simulink model "hybrid_controller_old3"  (R2024b)
settings: Solver=VariableStepAuto  StartTime=0.0  StopTime=20  RelTol=1e-3
undefined symbols (not defined in the file or in its folder): extractTop2x2, non_linear_m, non_linear_vcfg, wall_surface
libraries: roblocks x10

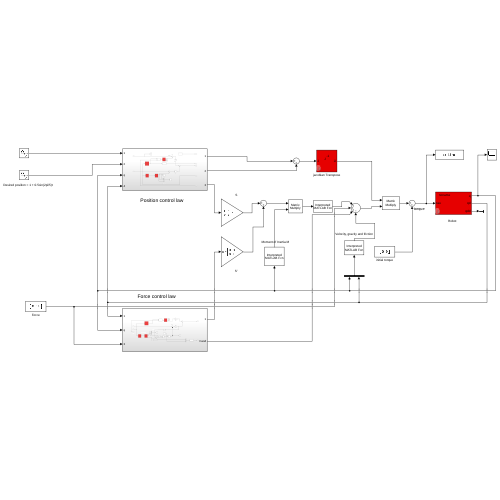
[thumbnail: Simulink's stored preview of the top-level diagram]
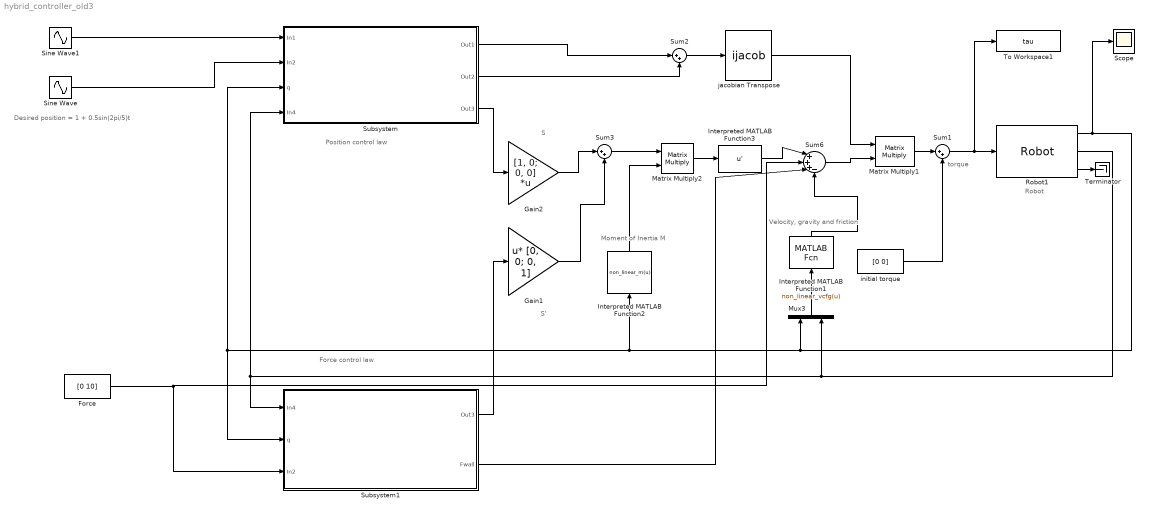
== system hybrid_controller_old3 ==
  note: Robot
  note: S
  note: Desired position = 1 + 0.5sin(2pi/5)t
  note: Position control law
  note: Moment of Inertia M
  note: Velocity, gravity and friction
  note: torque
  note: S'
  note: Force control law
  Force : Constant  Value=[0 10]
  Gain1 : Gain  Gain=[0, 0; 0, 1]  Multiplication=Matrix(u*K)
  Gain2 : Gain  Gain=[1, 0; 0, 0]  Multiplication=Matrix(K*u)
  Interpreted MATLAB Function1 : MATLABFcn  MATLABFcn=non_linear_vcfg(u)  OutputDimensions=[2 1]  Output1D=off
  Interpreted MATLAB Function2 : MATLABFcn  MATLABFcn=non_linear_m(u)  OutputDimensions=[2 2]  Output1D=off
  Interpreted MATLAB Function3 : MATLABFcn  MATLABFcn=u'  OutputDimensions=[2 1]  Output1D=off
  Matrix Multiply1 : Product  Multiplication=Matrix(*)
  Matrix Multiply2 : Product  Multiplication=Matrix(*)
  Mux3 : Mux  Inputs=2
  Robot1 : roblocks/Robot  robot=robot  q0=[0 0 0 0 0 0]
      link override Integrator: InitialCondition=[1 1]
      link override Integrator1: InitialCondition=[1 1]
  Scope : Scope
  Sine Wave : Sin  Amplitude=0.5  Bias=2.2  Frequency=1.256  SampleTime=0
  Sine Wave1 : Sin  Amplitude=0.28  Frequency=1.256  SampleTime=0
  Subsystem : Subsystem
  Subsystem1 : Subsystem
  Sum1 : Sum  Inputs=|++
  Sum2 : Sum  Inputs=|++
  Sum3 : Sum  Inputs=|++
  Sum6 : Sum  Inputs=|+++-
  Terminator : Terminator
  To Workspace1 : ToWorkspace  VariableName=tau  SampleTime=-1
      settings: Save2DSignal=2-D array (concatenate along first dimension)
  initial torque : Constant  Value=[0 0]
  jacobian Transpose : roblocks/ijacob
      link override inverse jacobian: MATLABFcn=u'
  wires:
  Interpreted MATLAB Function3/1 -> Sum6/1
  Robot1/2 -> Subsystem/4(In4), Subsystem1/1(In4), Mux3/2
  Robot1/1 -> Scope/1, Subsystem/3(q), Subsystem1/2(q), Interpreted MATLAB Function2/1, Mux3/1
  initial torque/1 -> Sum1/2
  Sum6/1 -> Matrix Multiply1/2
  jacobian Transpose/1 -> Matrix Multiply1/1
  Interpreted MATLAB Function2/1 -> Matrix Multiply2/2
  Matrix Multiply2/1 -> Interpreted MATLAB Function3/1
  Mux3/1 -> Interpreted MATLAB Function1/1
  Robot1/3 -> Terminator/1
  Matrix Multiply1/1 -> Sum1/1
  Sum1/1 -> Robot1/1, To Workspace1/1
  Sum2/1 -> jacobian Transpose/1
  Sine Wave1/1 -> Subsystem/1(In1)
  Sine Wave/1 -> Subsystem/2(In2)
  Subsystem/1(Out1) -> Sum2/1
  Subsystem/2(Out2) -> Sum2/2
  Subsystem/3(Out3) -> Gain2/1
  Gain2/1 -> Sum3/1
  Sum3/1 -> Matrix Multiply2/1
  Gain1/1 -> Sum3/2
  Force/1 -> Subsystem1/3(In2), Sum6/2
  Interpreted MATLAB Function1/1 -> Sum6/4
  Subsystem1/2(Fwall) -> Sum6/3
  Subsystem1/1(Out3) -> Gain1/1

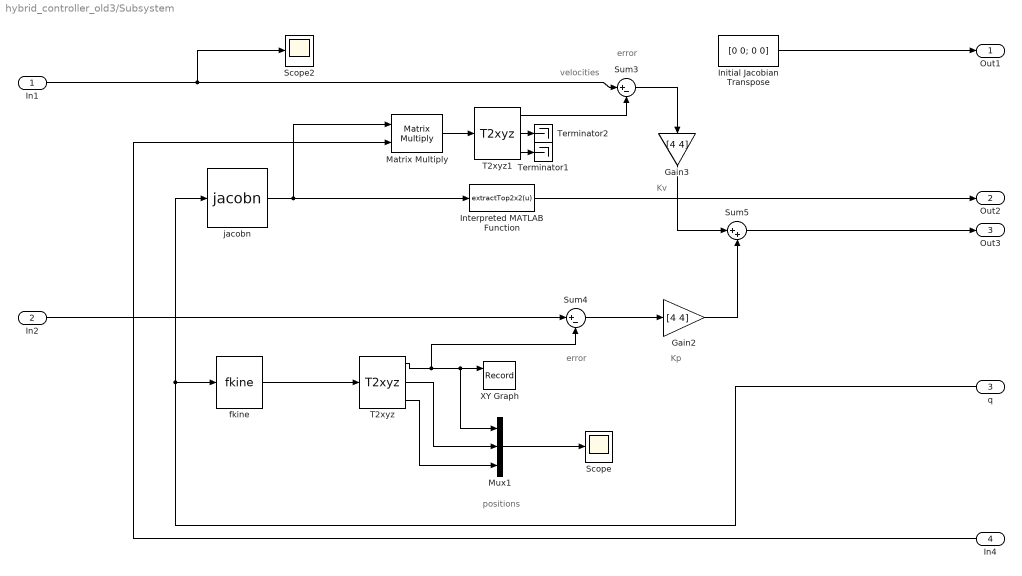
== system hybrid_controller_old3/Subsystem ==
  note: Kv
  note: error
  note: velocities
  note: error
  note: Kp
  note: positions
  In1 : Inport
  In2 : Inport  Port=2
  q : Inport  Port=3
  In4 : Inport  Port=4
  Gain2 : Gain  Gain=[4 4]
  Gain3 : Gain  Gain=[4 4]
  Initial Jacobian Transpose : Constant  Value=[0 0; 0 0]
  Interpreted MATLAB Function : MATLABFcn  MATLABFcn=extractTop2x2(u)  OutputDimensions=[2 2]  Output1D=off
  Matrix Multiply : Product  Multiplication=Matrix(*)
  Mux1 : Mux  Inputs=3
  Scope : Scope
  Scope2 : Scope
  Sum3 : Sum  Inputs=|+-
  Sum4 : Sum  Inputs=|+-
  Sum5 : Sum  Inputs=|++
  T2xyz : roblocks/T2xyz
  T2xyz1 : roblocks/T2xyz
      link override MATLAB Fcn: MATLABFcn=transljac(u)
  Terminator1 : Terminator
  Terminator2 : Terminator
  XY Graph : Record  FileSettingsInternal="{\"entries\":[{\"content\":{\"excelSettings\":{\"content\":{},\"type\":\"Streamout.ExcelSettings\"}},\"type\":\"Streamout.FileSettingStorage\",\"uuid\":\"\"}],\"packageUris\":[\"http:\\/\\/schema.mathworks.com\\/mf0\\/streamout_blocks\\/R2020a\"],\"version\":\"1.0\"}"  Layout=[1 1]  SignalsInternal="{\"entries\":[{\"content\":{\"signals\":[{\"content\":{\"blockPath\":[],\"dimensions\":[1],\"domain\":\"\",\"lineColor\":\"#a2142f\",\"plots\":[ 1 ],\"port\":1,\"sid\":[\"\"],\"signalID\":1,\"signalName\":\"T2xyz:1\"},\"type\":\"RecordBlkView.Signal\",\"uuid\":\"\"},{\"content\":{\"blockPath\":[],\"dimensions\":[1],\"domain\":\"\",\"lineColor\":\"#139fff\",\"plots\":[ 1 ],\"port\":2,\"sid\":[\"\"],\"signalID\":2},\"type\":\"RecordBlkView.Signal\",\"uuid\":\"\"}]},\"type\":\"RecordBlkView.InputSignals\",\"uuid\":\"\"}],\"packageUris\":[\"http:\\/\\/schema.mathworks.com\\/mf0\\/streamout_blocks\\/R2020a\"],\"version\":\"1.0\"}"  VisualizationBindings="{\"xyplotplugin\":{\"info\":[{\"series\":[{\"bindingParametersList\":[{\"parameter\":\"X-Axis\",\"signalID\":1,\"signalName\":\"T2xyz:1\"},{\"parameter\":\"Y-Axis\",\"signalID\":2,\"signalName\":\"XY Graph:2\"}],\"seriesID\":0}],\"subplotID\":1}]}}"  CompatibilityTag=XY
  fkine : roblocks/fkine  robot=robot
  jacobn : roblocks/jacobn  robot=robot
      link override MATLAB Fcn: MATLABFcn=jacobn(robot,u)
  Out1 : Outport
  Out2 : Outport  Port=2
  Out3 : Outport  Port=3
  wires:
  Interpreted MATLAB Function/1 -> Out2/1
  In4/1 -> Matrix Multiply/2
  Initial Jacobian Transpose/1 -> Out1/1
  Mux1/1 -> Scope/1
  T2xyz1/1 -> Sum3/2
  Gain3/1 -> Sum5/1
  fkine/1 -> T2xyz/1
  T2xyz/1 -> Sum4/2, XY Graph/1, Mux1/1
  Gain2/1 -> Sum5/2
  jacobn/1 -> Interpreted MATLAB Function/1, Matrix Multiply/1
  Sum5/1 -> Out3/1
  Sum3/1 -> Gain3/1
  Sum4/1 -> Gain2/1
  q/1 -> jacobn/1, fkine/1
  In1/1 -> Scope2/1, Sum3/1
  Matrix Multiply/1 -> T2xyz1/1
  In2/1 -> Sum4/1
  T2xyz1/3 -> Terminator1/1
  T2xyz/2 -> Mux1/2
  T2xyz/3 -> Mux1/3
  T2xyz1/2 -> Terminator2/1

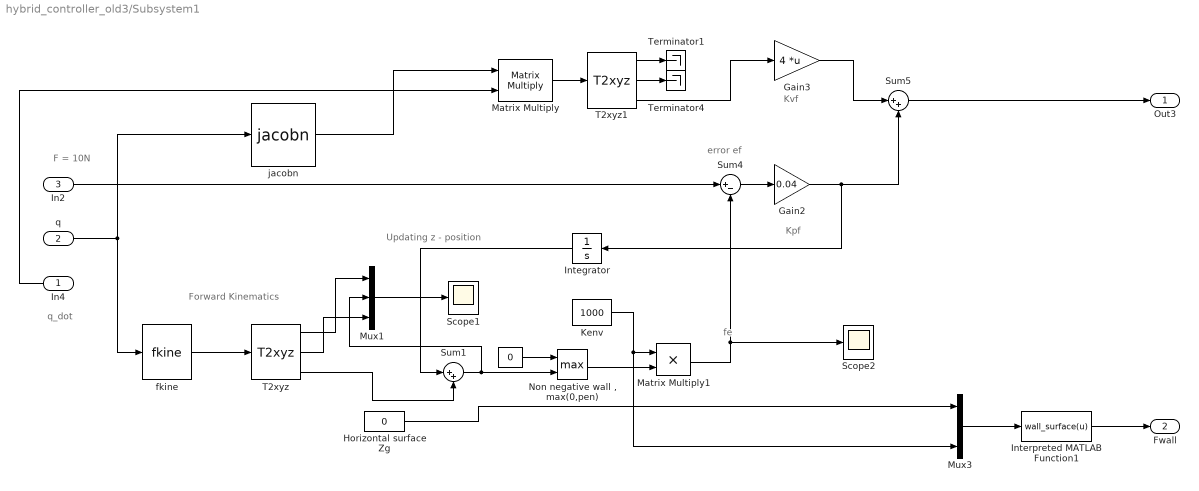
== system hybrid_controller_old3/Subsystem1 ==
  note: Updating z - position
  note: Forward Kinematics
  note: F = 10N
  note: q_dot
  note: Kvf
  note: error ef
  note: Kpf
  note: fe
  In4 : Inport
  q : Inport  Port=2
  In2 : Inport  Port=3
  " " : Constant  Value=0
  " Horizontal surface Zg" : Constant  Value=0
  " Kenv" : Constant  Value=1000
  Gain2 : Gain  Gain=0.04
  Gain3 : Gain  Gain=4  Multiplication=Matrix(K*u)
  Integrator : Integrator
  Interpreted MATLAB Function1 : MATLABFcn  MATLABFcn=wall_surface(u)  OutputDimensions=[2 1]  Output1D=off
  Matrix Multiply : Product  Multiplication=Matrix(*)
  Matrix Multiply1 : Product
  Mux1 : Mux  Inputs=3
  Mux3 : Mux  Inputs=3
  "Non negative wall , max(0,pen)" : MinMax  Function=max  Inputs=2
  Scope1 : Scope
  Scope2 : Scope
  Sum1 : Sum  Inputs=|++
  Sum4 : Sum  Inputs=|+-
  Sum5 : Sum  Inputs=|++
  T2xyz : roblocks/T2xyz
  T2xyz1 : roblocks/T2xyz
      link override MATLAB Fcn: MATLABFcn=transljac(u)
  Terminator1 : Terminator
  Terminator4 : Terminator
  fkine : roblocks/fkine  robot=robot
  jacobn : roblocks/jacobn  robot=robot
      link override MATLAB Fcn: MATLABFcn=jacobn(robot,u)
  Out3 : Outport
  Fwall : Outport  Port=2
  wires:
  In4/1 -> Matrix Multiply/2
  Gain3/1 -> Sum5/1
  Gain2/1 -> Integrator/1, Sum5/2
  jacobn/1 -> Matrix Multiply/1
  Sum5/1 -> Out3/1
  q/1 -> jacobn/1, fkine/1
  Matrix Multiply/1 -> T2xyz1/1
  In2/1 -> Sum4/1
  T2xyz1/2 -> Terminator4/1
  T2xyz/1 -> Mux1/1
  " Horizontal surface Zg"/1 -> Mux3/1
  Sum4/1 -> Gain2/1
  " Kenv"/1 -> Matrix Multiply1/1, Mux3/3
  Mux1/1 -> Scope1/1
  Matrix Multiply1/1 -> Sum4/2, Scope2/1
  Interpreted MATLAB Function1/1 -> Fwall/1
  fkine/1 -> T2xyz/1
  Mux3/1 -> Interpreted MATLAB Function1/1
  T2xyz/3 -> Sum1/2
  T2xyz1/3 -> Gain3/1
  T2xyz1/1 -> Terminator1/1
  Integrator/1 -> Sum1/1
  " "/1 -> "Non negative wall , max(0,pen)"/1
  "Non negative wall , max(0,pen)"/1 -> Matrix Multiply1/2
  Sum1/1 -> Mux1/2, "Non negative wall , max(0,pen)"/2
  T2xyz/2 -> Mux1/3
